simulink model "P_model"  (R2022b)
settings: Solver=VariableStepAuto  StartTime=0.0  StopTime=10  RelTol=1e-3
undefined symbols (not defined in the file): J, ke, km, kp, L, R, target, Umin
settings Model: Creator=khanh  LastModifiedBy=anton

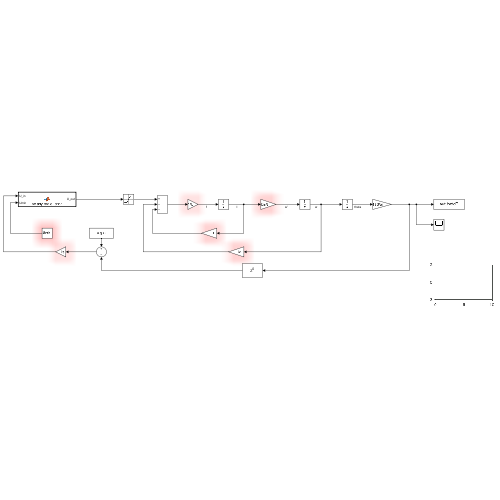
[thumbnail: Simulink's stored preview of the top-level diagram]
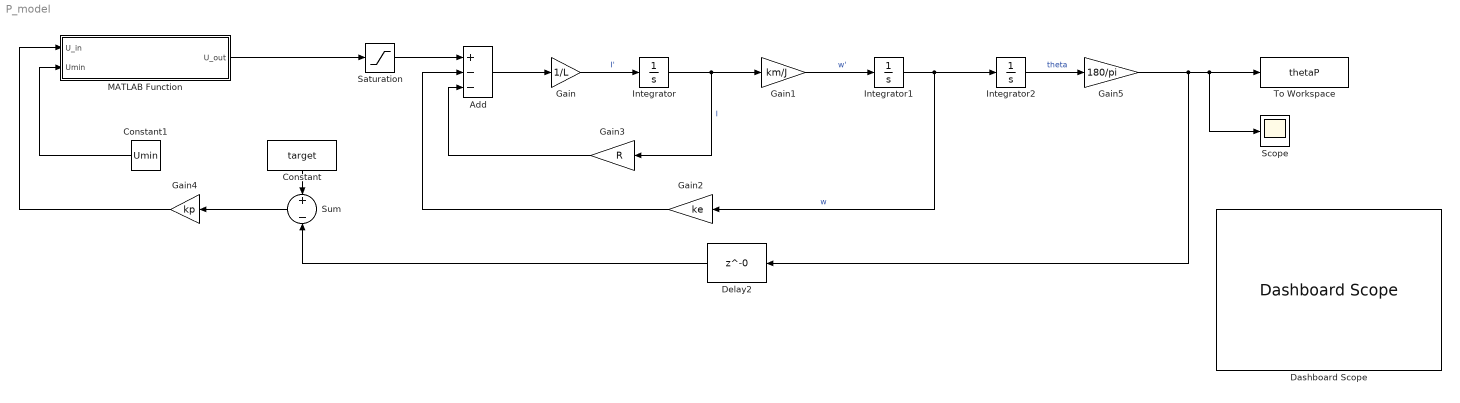
== system P_model ==
  Add : Sum  Inputs=+--
  Constant : Constant  Value=target
  Constant1 : Constant  Value=Umin
  Dashboard Scope : DashboardScope
  Delay2 : Delay  DelayLength=0  InitialCondition=0  SampleTime=50e-6
  Gain : Gain  Gain=1/L
  Gain1 : Gain  Gain=km/J
  Gain2 : Gain  Gain=ke
  Gain3 : Gain  Gain=R
  Gain4 : Gain  Gain=kp
  Gain5 : Gain  Gain=180/pi
  Integrator : Integrator
  Integrator1 : Integrator
  Integrator2 : Integrator
  MATLAB Function : MATLAB Function  TreatAsAtomicUnit=on
  Saturation : Saturate  UpperLimit=8.05  LowerLimit=-8.05
  Scope : Scope
  Sum : Sum  Inputs=+-
  To Workspace : ToWorkspace  VariableName=thetaP  SaveFormat=Timeseries  SampleTime=-1
  wires:
  Saturation/1 -> Add/1
  Add/1 -> Gain/1
  Gain/1 -> Integrator/1  "I'"
  Integrator/1 -> Gain3/1, Gain1/1  "I"
  Gain1/1 -> Integrator1/1  "w'"
  Integrator1/1 -> Gain2/1, Integrator2/1  "w"
  Gain2/1 -> Add/2
  Gain3/1 -> Add/3
  Constant/1 -> Sum/1
  Gain4/1 -> MATLAB Function/1(U_in)
  Sum/1 -> Gain4/1
  Constant1/1 -> MATLAB Function/2(Umin)
  MATLAB Function/1(U_out) -> Saturation/1
  Integrator2/1 -> Gain5/1  "theta"
  Gain5/1 -> Delay2/1, Scope/1, To Workspace/1
  Delay2/1 -> Sum/2

== matlab function P_model/MATLAB Function ==
  data: U_out output; U_in input; Umin input
function U_out = steady_state_error(U_in, Umin)
    if (abs(U_in) < Umin)
        U_out = 0;
    else
        U_out = U_in;
    end

end
